simulink model "Main_Model"  (R2022b)
settings: Solver=VariableStepAuto  StartTime=0.0  StopTime=2  FixedStep=1e-4  RelTol=1e-6
InitFcn:
  | Lfg=1.75e-3;
  | Lfc=3.5e-3;
  | Lf = Lfg +Lfc;
  | Cf=20e-6;
  | 
  | Lg=0.0035;
  | L=Lf+Lg;
  | Rg=0.5498*2;
  | k=0.707;
  | omega0 = 100*pi;
  | kp1=10;
  | ki1=250;
  | %kp1=10;
  | %ki1=250;
  | kp2=10;
  | ki2=250;
undefined symbols (not defined in the file): den_Tn2p_11, den_Tn2p_12, den_Tp2n_11, den_Tp2n_12, num_Tn2p_11, num_Tn2p_12, num_Tp2n_11, num_Tp2n_12
libraries: spsSeriesRLCBranchLib x12, slpidlib x9, spsControlledVoltageSourceLib x6, spsThreePhaseVIMeasurementLib x3, spsAlphaBetaZerotoabcLib x2, simulink x2, spsGroundLib x1, spspowerguiLib x1
(part 2 of 2)

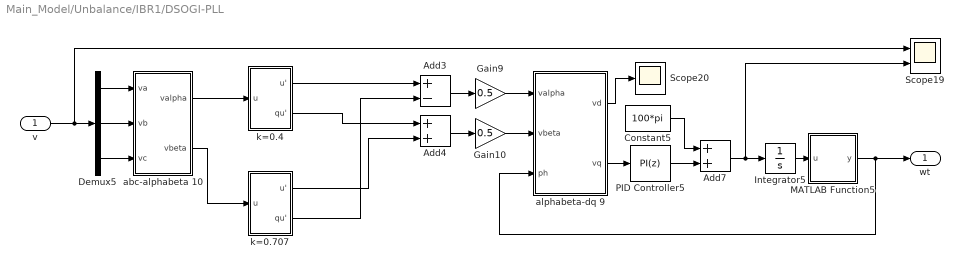
== system Main_Model/Unbalance/IBR1/DSOGI-PLL ==
  v : Inport
  Add3 : Sum  Inputs=+-
  Add4 : Sum
  Add7 : Sum
  Constant5 : Constant  Value=100*pi
  Demux5 : Demux  Outputs=3
  Gain10 : Gain  Gain=0.5
  Gain9 : Gain  Gain=0.5
  Integrator5 : Integrator
  MATLAB Function5 : MATLAB Function  TreatAsAtomicUnit=on
  PID Controller5 : slpidlib/PID Controller  Controller=PI  Form=Parallel  TimeDomain=Discrete-time  UseExternalTs=off  SampleTime=-1  IntegratorMethod=Forward Euler  FilterMethod=Forward Euler  ControllerParametersSource=internal  P=1  I=3  UseKiTs=off  D=0  N=100  UseFilter=on  TunerSelectOption=Transfer Function Based (PID Tuner App)  InitialConditionSource=internal  InitialConditionForIntegrator=0  InitialConditionForFilter=0  DifferentiatorICPrevScaledInput=0  ExternalReset=none  TrackingMode=off  Kt=1  LimitOutput=off  SatLimitsSource=internal  UpperSaturationLimit=inf  LowerSaturationLimit=-inf  LinearizeAsGain=on  AntiWindupMode=none  Kb=1  LimitIntegrator=off  UpperIntegratorSaturationLimit=inf  LowerIntegratorSaturationLimit=-inf  POutMin=[]  POutMax=[]  IOutMin=[]  IOutMax=[]  DOutMin=[]  DOutMax=[]  NOutMin=[]  NOutMax=[]  SumOutMin=[]  SumOutMax=[]  SaturationOutMin=[]  SaturationOutMax=[]  PParamMin=[]  PParamMax=[]  IParamMin=[]  IParamMax=[]  DParamMin=[]  DParamMax=[]  NParamMin=[]  NParamMax=[]  KbParamMin=[]  KbParamMax=[]  KtParamMin=[]  KtParamMax=[]  KbOutMin=[]  KbOutMax=[]  KtOutMin=[]  KtOutMax=[]  IntegratorOutMin=[]  IntegratorOutMax=[]  FilterOutMin=[]  FilterOutMax=[]  SumI1OutMin=[]  SumI1OutMax=[]  SumI2OutMin=[]  SumI2OutMax=[]  SumI3OutMin=[]  SumI3OutMax=[]  SumI4OutMin=[]  SumI4OutMax=[]  SumDOutMin=[]  SumDOutMax=[]  DifferentiatorOutMin=[]  DifferentiatorOutMax=[]  FilterDiffOutCoefMin=[]  FilterDiffOutCoefMax=[]  ReciprocalOutMin=[]  ReciprocalOutMax=[]  SumDenOutMin=[]  SumDenOutMax=[]  SumNumOutMin=[]  SumNumOutMax=[]  DivideOutMin=[]  DivideOutMax=[]  UdiffTsProdOutMin=[]  UdiffTsProdOutMax=[]  NTsProdOutMin=[]  NTsProdOutMax=[]  UintegralTsProdOutMin=[]  UintegralTsProdOutMax=[]  UngainTsProdOutMin=[]  UngainTsProdOutMax=[]  ClampingZeroOutDataTypeStr=Inherit: Inherit via back propagation  ClampingZeroOutMin=[]  ClampingZeroOutMax=[]  FilterDenConstantOutDataTypeStr=Inherit: Inherit via back propagation  FilterDenConstantOutMin=[]  FilterDenConstantOutMax=[]  PCopyOutDataTypeStr=Inherit: Inherit via back propagation  PCopyOutMin=[]  PCopyOutMax=[]  NCopyOutDataTypeStr=Inherit: Inherit via back propagation  NCopyOutMin=[]  NCopyOutMax=[]  IntegratorContinuousStateAttributes=''  IntegratorStateMustResolveToSignalObject=off  IntegratorRTWStateStorageClass=Auto  FilterContinuousStateAttributes=''  FilterStateMustResolveToSignalObject=off  FilterRTWStateStorageClass=Auto  ParallelPVariant=InternalParameters  IdealPVariant=Disabled  IVariant=InternalParameters  DVariant=Disabled  IntegratorVariant=Discrete  SatVariant=Disabled  AWVariant=Passthrough  PCopyVariant=Disabled  TRVariant=Disabled  FdbkBlocksVariant=Forward  IdealPFdbkVariant=Disabled  SatFdbkVariant=Disabled  DerivativeFilterVariant=Disabled  NVariant=Disabled  NCopyVariant=Disabled_SignalSpec  FilterICVariant=Disabled  IntegratorICVariant=InternalICs  ExternalResetVariant=Disabled  TRSumVariant=Passthrough  SumFdbkVariant=Disabled  SumVariant=Sum_PI  TsampFilterVariant=InternalTs  TsampNgainVariant=Passthrough  TsampIntegralVariant=Passthrough  ExternalSaturationOutDataTypeStr=Inherit: Same as second input
  Scope19 : Scope  NumInputPorts=2
  Scope20 : Scope
  abc-alphabeta 10 : MATLAB Function  TreatAsAtomicUnit=on
  alphabeta-dq 9 : MATLAB Function  TreatAsAtomicUnit=on
  k=0.4 : Subsystem
  k=0.707 : Subsystem
  wt : Outport
  wires:
  Add7/1 -> Integrator5/1, Scope19/2
  Constant5/1 -> Add7/1
  Demux5/1 -> abc-alphabeta 10/1(va)
  Gain9/1 -> alphabeta-dq 9/1(valpha)
  alphabeta-dq 9/1(vd) -> Scope20/1
  alphabeta-dq 9/2(vq) -> PID Controller5/1
  Gain10/1 -> alphabeta-dq 9/2(vbeta)
  Demux5/2 -> abc-alphabeta 10/2(vb)
  v/1 -> Demux5/1, Scope19/1
  Demux5/3 -> abc-alphabeta 10/3(vc)
  PID Controller5/1 -> Add7/2
  Integrator5/1 -> MATLAB Function5/1(u)
  MATLAB Function5/1(y) -> wt/1, alphabeta-dq 9/3(ph)
  Add4/1 -> Gain10/1
  k=0.4/2(qu') -> Add4/1
  k=0.707/2(qu') -> Add3/2
  k=0.4/1(u') -> Add3/1
  k=0.707/1(u') -> Add4/2
  Add3/1 -> Gain9/1
  abc-alphabeta 10/1(valpha) -> k=0.4/1(u)
  abc-alphabeta 10/2(vbeta) -> k=0.707/1(u)

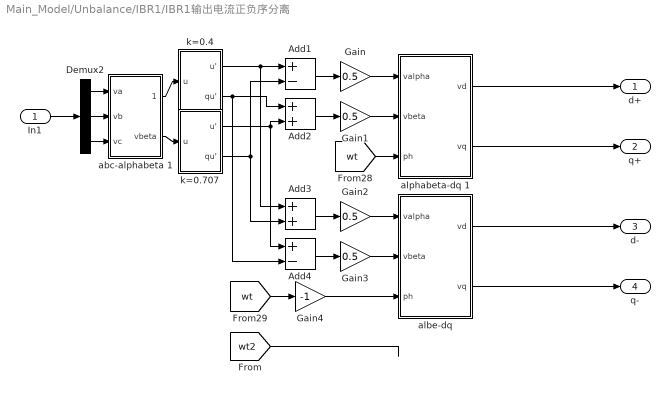
== system Main_Model/Unbalance/IBR1/IBR1输出电流正负序分离 ==
  In1 : Inport
  Add1 : Sum  Inputs=+-
  Add2 : Sum
  Add3 : Sum
  Add4 : Sum  Inputs=+-
  Demux2 : Demux  Outputs=3
  Gain{,1..3} (4 alike) : Gain  Gain=0.5
  Gain4 : Gain  Gain=-1
  abc-alphabeta 1 : MATLAB Function  TreatAsAtomicUnit=on
  albe-dq : MATLAB Function  TreatAsAtomicUnit=on
  alphabeta-dq 1 : MATLAB Function  TreatAsAtomicUnit=on
  k=0.4 : Subsystem
  k=0.707 : Subsystem
  d+ : Outport  VectorParamsAs1DForOutWhenUnconnected=off
  q+ : Outport  Port=2  VectorParamsAs1DForOutWhenUnconnected=off
  d- : Outport  Port=3  VectorParamsAs1DForOutWhenUnconnected=off
  q- : Outport  Port=4  VectorParamsAs1DForOutWhenUnconnected=off
  wires:
  Demux2/2 -> abc-alphabeta 1/2(vb)
  k=0.4/1(u') -> Add3/1, Add1/1
  k=0.707/1(u') -> Add2/2, Add4/1
  Add1/1 -> Gain/1
  Demux2/1 -> abc-alphabeta 1/1(va)
  Gain/1 -> alphabeta-dq 1/1(valpha)
  k=0.4/2(qu') -> Add2/1, Add4/2
  k=0.707/2(qu') -> Add3/2, Add1/2
  Add2/1 -> Gain1/1
  Add3/1 -> Gain2/1
  [wt] -> Gain4/1
  Gain1/1 -> alphabeta-dq 1/2(vbeta)
  In1/1 -> Demux2/1
  Gain2/1 -> albe-dq/1(valpha)
  Demux2/3 -> abc-alphabeta 1/3(vc)
  [wt] -> alphabeta-dq 1/3(ph)
  Gain4/1 -> albe-dq/3(ph)
  Add4/1 -> Gain3/1
  abc-alphabeta 1/2(vbeta) -> k=0.707/1(u)
  Gain3/1 -> albe-dq/2(vbeta)
  abc-alphabeta 1/1(valpha) -> k=0.4/1(u)
  alphabeta-dq 1/1(vd) -> d+/1
  alphabeta-dq 1/2(vq) -> q+/1
  albe-dq/1(vd) -> d-/1
  albe-dq/2(vq) -> q-/1
  [wt2] -> ?

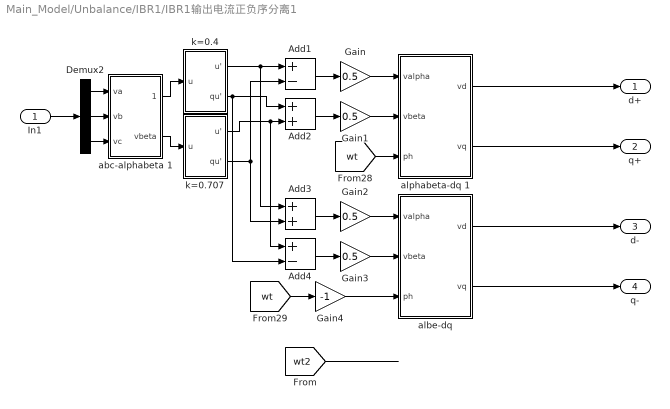
== system Main_Model/Unbalance/IBR1/IBR1输出电流正负序分离1 ==
  In1 : Inport
  Add1 : Sum  Inputs=+-
  Add2 : Sum
  Add3 : Sum
  Add4 : Sum  Inputs=+-
  Demux2 : Demux  Outputs=3
  Gain{,1..3} (4 alike) : Gain  Gain=0.5
  Gain4 : Gain  Gain=-1
  abc-alphabeta 1 : MATLAB Function  TreatAsAtomicUnit=on
  albe-dq : MATLAB Function  TreatAsAtomicUnit=on
  alphabeta-dq 1 : MATLAB Function  TreatAsAtomicUnit=on
  k=0.4 : Subsystem
  k=0.707 : Subsystem
  d+ : Outport  VectorParamsAs1DForOutWhenUnconnected=off
  q+ : Outport  Port=2  VectorParamsAs1DForOutWhenUnconnected=off
  d- : Outport  Port=3  VectorParamsAs1DForOutWhenUnconnected=off
  q- : Outport  Port=4  VectorParamsAs1DForOutWhenUnconnected=off
  wires:
  [wt2] -> ?
  albe-dq/2(vq) -> q-/1
  albe-dq/1(vd) -> d-/1
  alphabeta-dq 1/2(vq) -> q+/1
  alphabeta-dq 1/1(vd) -> d+/1
  abc-alphabeta 1/1(valpha) -> k=0.4/1(u)
  Gain3/1 -> albe-dq/2(vbeta)
  abc-alphabeta 1/2(vbeta) -> k=0.707/1(u)
  Add4/1 -> Gain3/1
  Gain4/1 -> albe-dq/3(ph)
  [wt] -> alphabeta-dq 1/3(ph)
  Demux2/3 -> abc-alphabeta 1/3(vc)
  Gain2/1 -> albe-dq/1(valpha)
  In1/1 -> Demux2/1
  Gain1/1 -> alphabeta-dq 1/2(vbeta)
  [wt] -> Gain4/1
  Add3/1 -> Gain2/1
  Add2/1 -> Gain1/1
  k=0.707/2(qu') -> Add3/2, Add1/2
  k=0.4/2(qu') -> Add4/2, Add2/1
  Gain/1 -> alphabeta-dq 1/1(valpha)
  Demux2/1 -> abc-alphabeta 1/1(va)
  Add1/1 -> Gain/1
  k=0.707/1(u') -> Add2/2, Add4/1
  k=0.4/1(u') -> Add1/1, Add3/1
  Demux2/2 -> abc-alphabeta 1/2(vb)

== system Main_Model/Unbalance/Grid/negative_sequence_dq>>abc4/dq0>>alpha_beta_0 ==
  alpha_beta_0 : Inport
  Gain3 : Gain  Gain="[ 1   0   1; -1/2  sqrt(3)/2   1; -1/2  -sqrt(3)/2  1 ]"  Multiplication=Matrix(K*u) (u vector)  SaturateOnIntegerOverflow=on  OutDataTypeStr=Inherit: Same as input  ParamDataTypeStr=Inherit: Same as input
  abc : Outport
  wires:
  alpha_beta_0/1 -> Gain3/1
  Gain3/1 -> abc/1

== system Main_Model/Unbalance/Grid/positive_sequence_dq>>abc1/dq0>>alpha_beta_0 ==
  alpha_beta_0 : Inport
  Gain3 : Gain  Gain="[ 1   0   1; -1/2  sqrt(3)/2   1; -1/2  -sqrt(3)/2  1 ]"  Multiplication=Matrix(K*u) (u vector)  SaturateOnIntegerOverflow=on  OutDataTypeStr=Inherit: Same as input  ParamDataTypeStr=Inherit: Same as input
  abc : Outport
  wires:
  alpha_beta_0/1 -> Gain3/1
  Gain3/1 -> abc/1

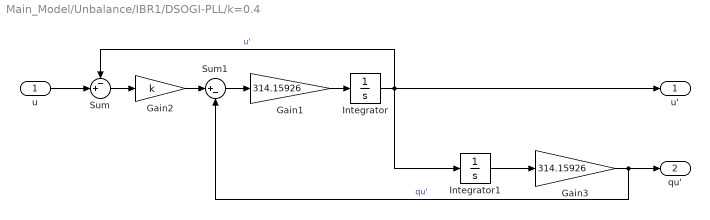
== system Main_Model/Unbalance/IBR1/DSOGI-PLL/k=0.4 ==
  u : Inport
  Gain1 : Gain  Gain=314.15926
  Gain2 : Gain  Gain=k
  Gain3 : Gain  Gain=314.15926
  Integrator : Integrator
  Integrator1 : Integrator
  Sum : Sum  Inputs=-+|
  Sum1 : Sum  Inputs=|+-
  u' : Outport
  qu' : Outport  Port=2
  wires:
  Sum/1 -> Gain2/1
  Gain3/1 -> Sum1/2, qu'/1  "qu'"
  Integrator1/1 -> Gain3/1
  Gain2/1 -> Sum1/1
  Integrator/1 -> Sum/1, u'/1, Integrator1/1  "u'"
  u/1 -> Sum/2
  Sum1/1 -> Gain1/1
  Gain1/1 -> Integrator/1

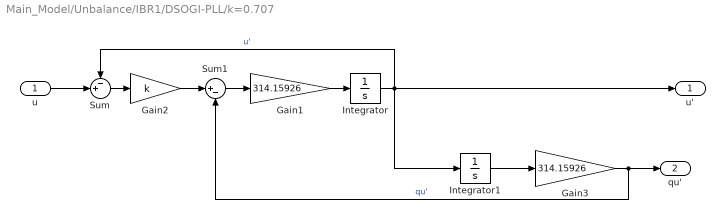
== system Main_Model/Unbalance/IBR1/DSOGI-PLL/k=0.707 ==
  u : Inport
  Gain1 : Gain  Gain=314.15926
  Gain2 : Gain  Gain=k
  Gain3 : Gain  Gain=314.15926
  Integrator : Integrator
  Integrator1 : Integrator
  Sum : Sum  Inputs=-+|
  Sum1 : Sum  Inputs=|+-
  u' : Outport
  qu' : Outport  Port=2
  wires:
  Sum/1 -> Gain2/1
  Gain3/1 -> Sum1/2, qu'/1  "qu'"
  Integrator1/1 -> Gain3/1
  Gain2/1 -> Sum1/1
  Integrator/1 -> Sum/1, u'/1, Integrator1/1  "u'"
  u/1 -> Sum/2
  Sum1/1 -> Gain1/1
  Gain1/1 -> Integrator/1

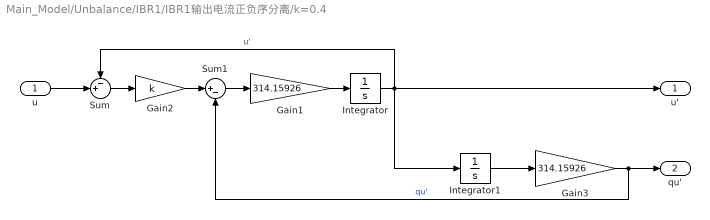
== system Main_Model/Unbalance/IBR1/IBR1输出电流正负序分离/k=0.4 ==
  u : Inport
  Gain1 : Gain  Gain=314.15926
  Gain2 : Gain  Gain=k
  Gain3 : Gain  Gain=314.15926
  Integrator : Integrator
  Integrator1 : Integrator
  Sum : Sum  Inputs=-+|
  Sum1 : Sum  Inputs=|+-
  u' : Outport
  qu' : Outport  Port=2
  wires:
  Sum/1 -> Gain2/1
  Gain3/1 -> Sum1/2, qu'/1  "qu'"
  Integrator1/1 -> Gain3/1
  Gain2/1 -> Sum1/1
  Integrator/1 -> Sum/1, u'/1, Integrator1/1  "u'"
  u/1 -> Sum/2
  Sum1/1 -> Gain1/1
  Gain1/1 -> Integrator/1

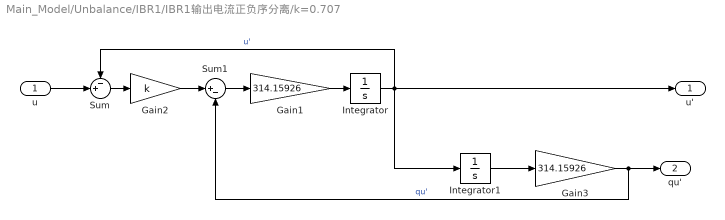
== system Main_Model/Unbalance/IBR1/IBR1输出电流正负序分离/k=0.707 ==
  u : Inport
  Gain1 : Gain  Gain=314.15926
  Gain2 : Gain  Gain=k
  Gain3 : Gain  Gain=314.15926
  Integrator : Integrator
  Integrator1 : Integrator
  Sum : Sum  Inputs=-+|
  Sum1 : Sum  Inputs=|+-
  u' : Outport
  qu' : Outport  Port=2
  wires:
  Sum/1 -> Gain2/1
  Gain3/1 -> Sum1/2, qu'/1  "qu'"
  Integrator1/1 -> Gain3/1
  Gain2/1 -> Sum1/1
  Integrator/1 -> Sum/1, u'/1, Integrator1/1  "u'"
  u/1 -> Sum/2
  Sum1/1 -> Gain1/1
  Gain1/1 -> Integrator/1

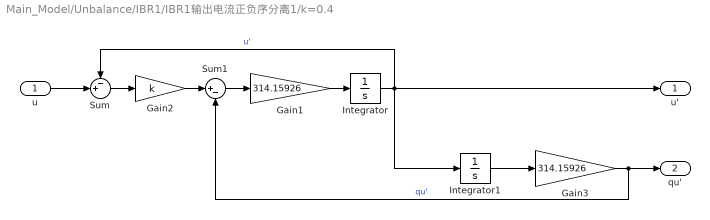
== system Main_Model/Unbalance/IBR1/IBR1输出电流正负序分离1/k=0.4 ==
  u : Inport
  Gain1 : Gain  Gain=314.15926
  Gain2 : Gain  Gain=k
  Gain3 : Gain  Gain=314.15926
  Integrator : Integrator
  Integrator1 : Integrator
  Sum : Sum  Inputs=-+|
  Sum1 : Sum  Inputs=|+-
  u' : Outport
  qu' : Outport  Port=2
  wires:
  Gain1/1 -> Integrator/1
  Sum1/1 -> Gain1/1
  u/1 -> Sum/2
  Integrator/1 -> Integrator1/1, u'/1, Sum/1  "u'"
  Gain2/1 -> Sum1/1
  Integrator1/1 -> Gain3/1
  Gain3/1 -> qu'/1, Sum1/2  "qu'"
  Sum/1 -> Gain2/1

== system Main_Model/Unbalance/IBR1/IBR1输出电流正负序分离1/k=0.707 ==
  u : Inport
  Gain1 : Gain  Gain=314.15926
  Gain2 : Gain  Gain=k
  Gain3 : Gain  Gain=314.15926
  Integrator : Integrator
  Integrator1 : Integrator
  Sum : Sum  Inputs=-+|
  Sum1 : Sum  Inputs=|+-
  u' : Outport
  qu' : Outport  Port=2
  wires:
  Gain1/1 -> Integrator/1
  Sum1/1 -> Gain1/1
  u/1 -> Sum/2
  Integrator/1 -> Integrator1/1, u'/1, Sum/1  "u'"
  Gain2/1 -> Sum1/1
  Integrator1/1 -> Gain3/1
  Gain3/1 -> qu'/1, Sum1/2  "qu'"
  Sum/1 -> Gain2/1

== matlab function Main_Model/Unbalance/IBR1/IBR1 ==
  data: vcd_p input; Vc_p output; vcq_p input; vcd_n input; vcq_n input; Vc_n output; VUF output
function [Vc_p, Vc_n, VUF] = fcn(vcd_p, vcq_p, vcd_n, vcq_n)
Vc_p = sqrt(vcd_p^2 + vcq_p^2);
Vc_n = sqrt(vcd_n^2 + vcq_n^2);
VUF = Vc_n/Vc_p;

== matlab function Main_Model/Subsystem1/albe-dq1 ==
  data: valpha input; vd output; vbeta input; ph input; vq output
function [vd,vq] = fcn(valpha,vbeta,ph)
vd=cos(ph)*valpha+sin(ph)*vbeta;
vq=-sin(ph)*valpha+cos(ph)*vbeta;

== matlab function Main_Model/Subsystem1/MATLAB Function4 ==
  data: ud input; ua output; uq input; ub output; ph input
function [ua,ub]= fcn(ud,uq,ph)
ua=ud*cos(ph)-uq*sin(ph);
ub=ud*sin(ph)+uq*cos(ph);

== matlab function Main_Model/Unbalance/IBR1/DSOGI-PLL/MATLAB Function5 ==
  data: u input; y output
function y = fcn(u)
y = rem(u,2*pi);

== matlab function Main_Model/Unbalance/IBR1/DSOGI-PLL/abc-alphabeta 10 ==
  data: va input; valpha output; vb input; vc input; vbeta output
function [valpha,vbeta] = fcn(va,vb,vc)
valpha=(2/3)*(1*va-1/2*vb-1/2*vc);
vbeta=(2/3)*(0*va+sqrt(3)/2*vb-sqrt(3)/2*vc);

== matlab function Main_Model/Unbalance/IBR1/DSOGI-PLL/alphabeta-dq 9 ==
  data: valpha input; vd output; vbeta input; ph input; vq output
function [vd,vq] = fcn(valpha,vbeta,ph)
vd=cos(ph)*valpha+sin(ph)*vbeta;
vq=-sin(ph)*valpha+cos(ph)*vbeta;

== matlab function Main_Model/Subsystem1/albe-dq4 ==
  data: valpha input; vd output; vbeta input; ph input; vq output
function [vd,vq] = fcn(valpha,vbeta,ph)
vd=cos(ph)*valpha+sin(ph)*vbeta;
vq=-sin(ph)*valpha+cos(ph)*vbeta;

== matlab function Main_Model/Unbalance/IBR1/MATLAB Function1 ==
  data: ud input; ua output; uq input; ub output; ph input
function [ua,ub]= fcn(ud,uq,ph)
ua=ud*cos(ph)-uq*sin(ph);
ub=ud*sin(ph)+uq*cos(ph);

== matlab function Main_Model/Unbalance/IBR1/IBR1输出电流正负序分离1/abc-alphabeta 1 ==
  data: va input; valpha output; vb input; vc input; vbeta output
function [valpha,vbeta] = fcn(va,vb,vc)
valpha=(2/3)*(1*va-1/2*vb-1/2*vc);
vbeta=(2/3)*(0*va+sqrt(3)/2*vb-sqrt(3)/2*vc);
% 恒幅值变换

== matlab function Main_Model/Subsystem1/MATLAB Function5 ==
  data: u input; y output
function y = fcn(u)
y = rem(u,2*pi);

== matlab function Main_Model/Unbalance/IBR1/IBR1输出电流正负序分离1/albe-dq ==
  data: valpha input; vd output; vbeta input; ph input; vq output
function [vd,vq] = fcn(valpha,vbeta,ph)
vd=cos(ph)*valpha+sin(ph)*vbeta;
vq=-sin(ph)*valpha+cos(ph)*vbeta;

== matlab function Main_Model/Unbalance/Grid/negative_sequence_dq>>abc4/MATLAB Function ==
  data: d input; alpha output; q input; theta input; beta output
function [alpha,beta] = fcn(d,q,theta)
%#codegen
A=[cos(theta) sin(theta);
   -sin(theta) cos(theta);];
y = A*[d;q;];
alpha=y(1);
beta=y(2);

== matlab function Main_Model/Unbalance/IBR1/IBR1输出电流正负序分离1/alphabeta-dq 1 ==
  data: valpha input; vd output; vbeta input; ph input; vq output
function [vd,vq] = fcn(valpha,vbeta,ph)
vd=cos(ph)*valpha+sin(ph)*vbeta;
vq=-sin(ph)*valpha+cos(ph)*vbeta;

== matlab function Main_Model/Subsystem1/MATLAB Function2 ==
  data: ud input; ua output; uq input; ub output; ph input
function [ua,ub]= fcn(ud,uq,ph)
ua=ud*cos(ph)-uq*sin(ph);
ub=ud*sin(ph)+uq*cos(ph);

== matlab function Main_Model/Subsystem1/MATLAB Function3 ==
  data: ud input; ua output; uq input; ub output; ph input
function [ua,ub]= fcn(ud,uq,ph)
ua=ud*cos(ph)-uq*sin(ph);
ub=ud*sin(ph)+uq*cos(ph);

== matlab function Main_Model/Subsystem1/albe-dq2 ==
  data: valpha input; vd output; vbeta input; ph input; vq output
function [vd,vq] = fcn(valpha,vbeta,ph)
vd=cos(ph)*valpha+sin(ph)*vbeta;
vq=-sin(ph)*valpha+cos(ph)*vbeta;

== matlab function Main_Model/Subsystem1/albe-dq3 ==
  data: valpha input; vd output; vbeta input; ph input; vq output
function [vd,vq] = fcn(valpha,vbeta,ph)
vd=cos(ph)*valpha+sin(ph)*vbeta;
vq=-sin(ph)*valpha+cos(ph)*vbeta;

== matlab function Main_Model/Unbalance/IBR1/MATLAB Function5 ==
  data: u input; y output
function y = fcn(u)
y = rem(u,2*pi);

== matlab function Main_Model/Unbalance/IBR1/MATLAB Function4 ==
  data: ud input; ua output; uq input; ub output; ph input
function [ua,ub]= fcn(ud,uq,ph)
ua=ud*cos(ph)-uq*sin(ph);
ub=ud*sin(ph)+uq*cos(ph);

== matlab function Main_Model/Subsystem1/MATLAB Function1 ==
  data: ud input; ua output; uq input; ub output; ph input
function [ua,ub]= fcn(ud,uq,ph)
ua=ud*cos(ph)-uq*sin(ph);
ub=ud*sin(ph)+uq*cos(ph);

== matlab function Main_Model/Unbalance/Grid/positive_sequence_dq>>abc1/MATLAB Function ==
  data: d input; alpha output; q input; theta input; beta output
function [alpha,beta] = fcn(d,q,theta)
%#codegen
A=[cos(theta) -sin(theta);
   sin(theta) cos(theta);];
y = A*[d;q;];
alpha=y(1);
beta=y(2);
%alpha轴与A轴重合

== matlab function Main_Model/Unbalance/IBR1/IBR1输出电流正负序分离/abc-alphabeta 1 ==
  data: va input; valpha output; vb input; vc input; vbeta output
function [valpha,vbeta] = fcn(va,vb,vc)
valpha=(2/3)*(1*va-1/2*vb-1/2*vc);
vbeta=(2/3)*(0*va+sqrt(3)/2*vb-sqrt(3)/2*vc);
% 恒幅值变换

== matlab function Main_Model/Unbalance/IBR1/IBR1输出电流正负序分离/albe-dq ==
  data: valpha input; vd output; vbeta input; ph input; vq output
function [vd,vq] = fcn(valpha,vbeta,ph)
vd=cos(ph)*valpha+sin(ph)*vbeta;
vq=-sin(ph)*valpha+cos(ph)*vbeta;

== matlab function Main_Model/Unbalance/IBR1/IBR1输出电流正负序分离/alphabeta-dq 1 ==
  data: valpha input; vd output; vbeta input; ph input; vq output
function [vd,vq] = fcn(valpha,vbeta,ph)
vd=cos(ph)*valpha+sin(ph)*vbeta;
vq=-sin(ph)*valpha+cos(ph)*vbeta;

== matlab function Main_Model/Unbalance/IBR1/dq轴功率计算 ==
  data: vd_p input; P1 output; vq_p input; vd_n input; vq_n input; id_p input; iq_p input; id_n input; iq_n input; Q1 output; P_p output; P_n output; Q_p output; Q_n output
function [P1, Q1, P_p, P_n, Q_p, Q_n] = fcn(vd_p, vq_p, vd_n, vq_n, id_p, iq_p, id_n, iq_n)
P_p = 1.5*(vd_p*id_p + vq_p*iq_p);
P_n = 1.5*(vd_n*id_n + vq_n*iq_n);
Q_p = 1.5*(vq_p*id_p - vd_p*iq_p);
Q_n = 1.5*(vq_n*id_n - vd_n*iq_n);
P1 = 1.5*(vd_p*id_p + vq_p*iq_p + vd_n*id_n + vq_n*iq_n);
Q1 = 1.5*(vq_p*id_p - vd_p*iq_p + vq_n*id_n - vd_n*iq_n);

%1.5倍
